simulink model "Transpuesta"  (R2017a)
settings: Solver=VariableStepAuto  StartTime=0.0  StopTime=10.0  RelTol=1e-3
libraries: dspmtrx3 x1, instrumentlib x1
settings Model: Creator=LuisFernando  LastModifiedBy=LuisFernando

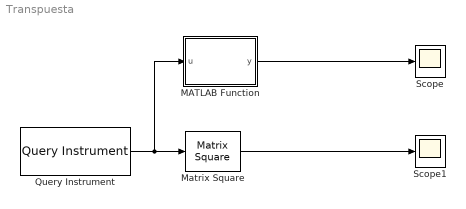
== system Transpuesta ==
  MATLAB Function : MATLAB Function  TreatAsAtomicUnit=on
  Matrix Square : dspmtrx3/Matrix Square  OutMin=[]  OutMax=[]
      settings: SourceProductName=DSP System Toolbox  SourceProductBaseCode=DS
  Query Instrument : instrumentlib/Query Instrument  sampleTime=inf  isWorkspaceObject=off  timeout=10  inputBufferSize=512  protocol=Serial  serialPort=COM2  baudRate=9600  gpibVendor=Agilent Technologies  boardIndex=0  primaryAddress=1  secondaryAddress=0  visaVendor=Agilent  visaSerialPort=0  chassisIndex=0  logicalAddress=0  tcpRemoteHost='127.0.0.1'  tcpRemotePort=4500  udpRemoteHost='127.0.0.1'  udpRemotePort=9090  visaTCPBoardIndex=0  visaTCPRemoteHost='127.0.0.1'  usbBoardIndex=0  usbManufID=0  usbModelCode=0  usbSerialNumber=0  initAction=None  initCommand='DATA:SOURCE CH1'  initFunction=get  queryCommand='curve?'  responseFormat=ASCII  asciiFormatting='%d,%d,%d'  precision=8-bit integer  byteOrder=Little endian  valuesToRead=1  removeBytes=off  afterOutputAction=Repeat query for new data  enableFrames=on  frameSize=3
      settings: SourceProductName=Instrument Control Toolbox  SourceProductBaseCode=IC
  Scope : Scope
  Scope1 : Scope
  wires:
  Query Instrument/1 -> MATLAB Function/1(u), Matrix Square/1
  MATLAB Function/1(y) -> Scope/1
  Matrix Square/1 -> Scope1/1

== matlab function Transpuesta/MATLAB Function ==
  data: u input; y output
function y = fcn(u)

y = u';
